simulink model "EV_mod"  (R2013b)
settings: Solver=ode1  StartTime=0.0  StopTime=tf  FixedStep=Ts  RelTol=1e-3
values from neighbouring files (symbols this model uses):
  A_Drag = 0.78    [EV_initial.m]
  Bat_Cap_Ah = 50    [EV_initial.m]
  eff_trans = 0.90    (= 0.9)    [EV_initial.m]
  f0 = 0.021    [EV_initial.m]
  f1 = 0    [EV_initial.m]
  f4 = 0    [EV_initial.m]
  g = 9.81    [EV_initial.m]
  Ki = 0.0    (= 0)    [EV_initial.m]
  Kp = 0.3    [EV_initial.m]
  m = m_Curb_WoBat_kg    (= 826)    [EV_initial.m]
  Mot_drive_n = [517 1021 2009 3247 4024 5025 6023 7017 8021 9008 10027]    [mod_tabs.mat]
  Mot_drive_ttq = [173.1 172 170.5 168.4 137.1 111.4 97.4 84.3 72.7 63.8 57.8]    [mod_tabs.mat]
  Mot_eff = [0.9093 0.9055 0.9401 0.9254 0.9287 0.9367 0.94 0.9292 0.9266 0.9191 0.8879 0.8947 ... (66 elements, 11x6)]    [mod_tabs.mat]
  R_f_charge = [0.0635340437122 0.0972918718458 0.105453801534 0.0989735084394 0.0862095416557 0.0738255704382 0.0918870144995 0.10417757919 0.0905696711114 0.0977276427179 0.0819350722889 0.155211698552 ... (16 elements, 1x16)]    [mod_tabs.mat]
  R_f_discharge = [0.12662204948 0.11936385128 0.118975090305 0.115399141433 0.117316920728 0.119061636403 0.1175114965 0.120632583027 0.128045365058 0.140195986159 0.137913717883 0.137947087219 ... (16 elements, 1x16)]    [mod_tabs.mat]
  r_gear = 9.34    [EV_initial.m]
  r_regen = 0.3    [EV_initial.m]
  SOC_f = [0.25 0.3 0.35 0.4 0.45 0.5 0.55 0.6 0.65 0.7 0.75 0.8 ... (16 elements, 1x16)]    [mod_tabs.mat]
  SOC_initial = 0.8    [EV_initial.m]
  T_brk_max = 800    [EV_initial.m]
  Uo_f_charge = [330.979042132 332.354241138 334.867975079 337.647567428 339.098272093 341.463293071 342.658764937 343.613546375 344.964982453 349.820174546 350.773879483 351.713350122 ... (16 elements, 1x16)]    [mod_tabs.mat]
  Uo_f_discharge = [329.578956913 331.264061644 334.222416797 335.977481552 337.118187606 339.421595672 340.30808504 340.898981164 343.01889846 346.179322896 346.685239696 346.505505514 ... (16 elements, 1x16)]    [mod_tabs.mat]
  v_init = v(1)/3.6    [EV_initial.m]
undefined symbols (not defined in the file): r_Wheel
libraries: simulink x1
settings Model: Creator=wanghonglei  LastModifiedBy=xinmei
settings DataIOCC: SignalLoggingSaveFormat=ModelDataLogs
settings OptimizationCC: ExpressionDepthLimit=2147483647
settings DebuggingCC: FcnCallInpInsideContextMsg=UseLocalSettings  StateNameClashWarn=warning
settings GRTTargetCC: CombineOutputUpdateFcns=off  GRTInterface=on

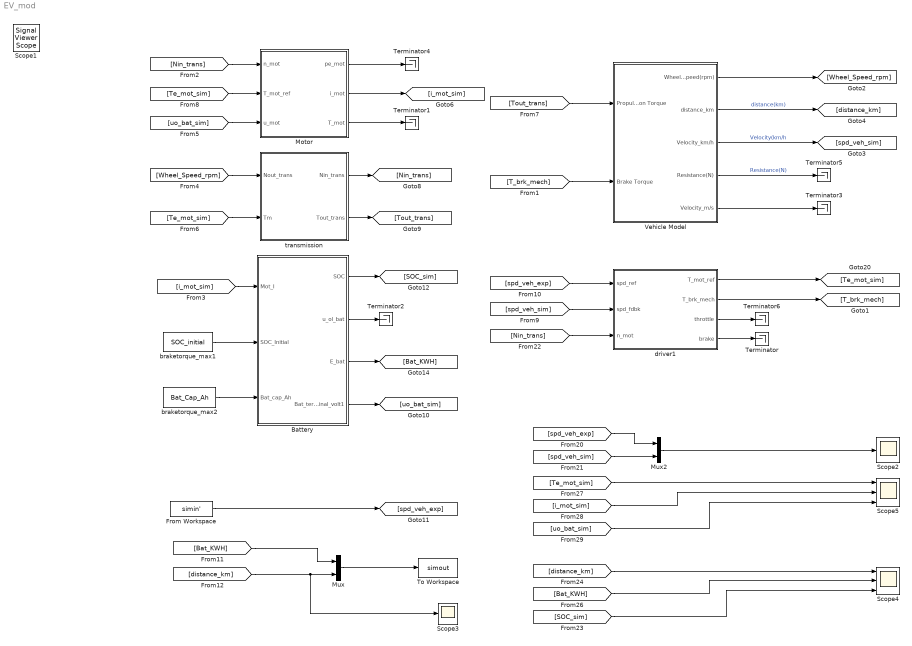
== system EV_mod ==
  Battery : Subsystem
  From Workspace : FromWorkspace  VariableName=simin'  SampleTime=0
  Motor : Subsystem
  Mux : Mux  Inputs=2
  Mux2 : Mux  Inputs=2
  Scope2 : Scope
  Scope3 : Scope
      settings: SaveName=ScopeData2
  Scope4 : Scope  NumInputPorts=3
      settings: YMin=-5~-5~-5  YMax=5~5~5  SaveName=ScopeData3
  Scope5 : Scope  NumInputPorts=3
      settings: YMin=-5~-5~-5  YMax=5~5~5
  Terminator{,1..6} (7 alike) : Terminator
  To Workspace : ToWorkspace  VariableName=simout  SampleTime=-1
      settings: MaxDataPoints=1
  Vehicle Model : Subsystem  mask{m=m, f0=f0, f1=f1, f4=f4, r=r_Wheel, A=0, K=0, g=g}
      mask prompts: m "Whole Vehicle Mass"; f0 "rolling resistant coefficient0"; f1 "rolling resistant coefficient1"; f4 "rolling resistant coefficient4"; r "radius"; A "Front Area"; K "wind resistant coeffcient"; g "Acceleration of Gravity"
  braketorque_max1 : Constant  Value=SOC_initial
  braketorque_max2 : Constant  Value=Bat_Cap_Ah
  driver1 : Subsystem
  transmission : Subsystem
  Scope1 : SignalViewerScope  IOType=viewer  NumInputPorts=4  LegendLocations=|  RefreshTime=0.035000
      | 633.2778      426.6944      187.6667         43.25
      | 712.2778      312.6944      108.6667         43.25
      | 640.2778      198.6944      180.6667         43.25
      | 640.2778      83.69444      180.6667         43.25
      settings: ShowLegends=on  TimeRange=450  YMin=0~-1~-20~-50  YMax=100~1~60~150
  wires:
  [T_brk_mech] -> Vehicle Model/2(Brake Torque)
  Vehicle Model/1(Wheel Speed(rpm)) -> [Wheel_Speed_rpm]
  [Wheel_Speed_rpm] -> transmission/1(Nout_trans)
  Vehicle Model/2(distance_km) -> [distance_km]  "distance(km)"
  transmission/1(Nin_trans) -> [Nin_trans]
  transmission/2(Tout_trans) -> [Tout_trans]
  [Tout_trans] -> Vehicle Model/1(Propulsion Torque)
  [i_mot_sim] -> Battery/1(Mot_I)
  braketorque_max1/1 -> Battery/2(SOC_Initial)
  braketorque_max2/1 -> Battery/3(Bat_cap_Ah)
  [Nin_trans] -> Motor/1(n_mot)
  Motor/2(i_mot) -> [i_mot_sim]
  [uo_bat_sim] -> Motor/3(u_mot)
  [Te_mot_sim] -> transmission/2(Tm)
  [Te_mot_sim] -> Motor/2(T_mot_ref)
  Battery/1(SOC) -> [SOC_sim]
  Battery/3(E_bat) -> [Bat_KWH]
  Battery/4(Bat_terminal_volt1) -> [uo_bat_sim]
  Battery/2(u_ol_bat) -> Terminator2/1
  Motor/1(pe_mot) -> Terminator4/1
  [spd_veh_exp] -> driver1/1(spd_ref)
  Vehicle Model/3(Velocity_km/h) -> [spd_veh_sim]  "Velocity(km/h"
  Vehicle Model/4(Resistance(N)) -> Terminator5/1  "Resistance(N)"
  Vehicle Model/5(Velocity_m/s) -> Terminator3/1
  From Workspace/1 -> [spd_veh_exp]
  [Bat_KWH] -> Mux/1
  [distance_km] -> Scope3/1, Mux/2
  Mux/1 -> To Workspace/1
  Mux2/1 -> Scope2/1
  [spd_veh_exp] -> Mux2/1
  [spd_veh_sim] -> Mux2/2
  [distance_km] -> Scope4/1
  [Bat_KWH] -> Scope4/2
  [SOC_sim] -> Scope4/3
  [Te_mot_sim] -> Scope5/1
  [i_mot_sim] -> Scope5/2
  [uo_bat_sim] -> Scope5/3
  [spd_veh_sim] -> driver1/2(spd_fdbk)
  [Nin_trans] -> driver1/3(n_mot)
  driver1/1(T_mot_ref) -> [Te_mot_sim]
  driver1/2(T_brk_mech) -> [T_brk_mech]
  driver1/3(throttle) -> Terminator6/1
  driver1/4(brake) -> Terminator/1
  Motor/3(T_mot) -> Terminator1/1

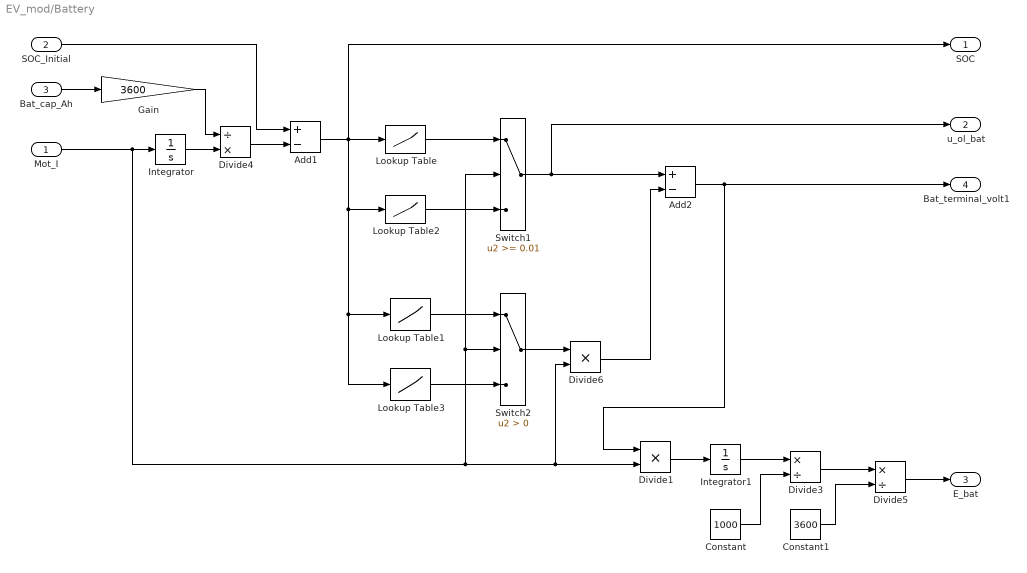
== system EV_mod/Battery ==
  Mot_I : Inport
  SOC_Initial : Inport  Port=2
  Bat_cap_Ah : Inport  Port=3
  Add1 : Sum  Inputs=+-
  Add2 : Sum  Inputs=+-
  Constant : Constant  Value=1000
  Constant1 : Constant  Value=3600
  Divide1 : Product  Inputs=**
  Divide3 : Product  Inputs=*/
  Divide4 : Product  Inputs=/*
  Divide5 : Product  Inputs=*/
  Divide6 : Product  Inputs=**
  Gain : Gain  Gain=3600
  Integrator : Integrator
  Integrator1 : Integrator
  Lookup Table : Lookup  InputValues=SOC_f  Table=Uo_f_discharge
  Lookup Table1 : Lookup  InputValues=SOC_f  Table=R_f_discharge
  Lookup Table2 : Lookup  InputValues=SOC_f  Table=Uo_f_charge
  Lookup Table3 : Lookup  InputValues=SOC_f  Table=R_f_charge
  Switch1 : Switch  Threshold=0.01
  Switch2 : Switch  Criteria=u2 > Threshold
  SOC : Outport
  u_ol_bat : Outport  Port=2
  E_bat : Outport  Port=3
  Bat_terminal_volt1 : Outport  Port=4
  wires:
  Bat_cap_Ah/1 -> Gain/1
  SOC_Initial/1 -> Add1/1
  Divide1/1 -> Integrator1/1
  Integrator1/1 -> Divide3/1
  Constant/1 -> Divide3/2
  Divide3/1 -> Divide5/1
  Constant1/1 -> Divide5/2
  Divide5/1 -> E_bat/1
  Divide6/1 -> Add2/2
  Add1/1 -> Lookup Table/1, Lookup Table3/1, Lookup Table1/1, Lookup Table2/1, SOC/1
  Switch2/1 -> Divide6/1
  Switch1/1 -> u_ol_bat/1, Add2/1
  Lookup Table/1 -> Switch1/1
  Lookup Table2/1 -> Switch1/3
  Mot_I/1 -> Switch2/2, Switch1/2, Divide6/2, Divide1/2, Integrator/1
  Lookup Table3/1 -> Switch2/3
  Lookup Table1/1 -> Switch2/1
  Add2/1 -> Bat_terminal_volt1/1, Divide1/1
  Integrator/1 -> Divide4/2
  Gain/1 -> Divide4/1
  Divide4/1 -> Add1/2

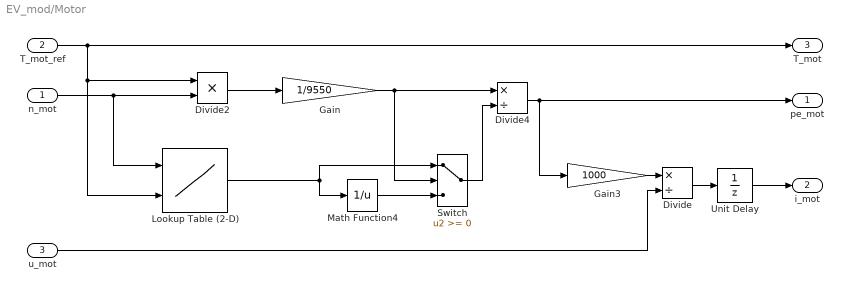
== system EV_mod/Motor ==
  n_mot : Inport
  T_mot_ref : Inport  Port=2
  u_mot : Inport  Port=3
  Divide : Product  Inputs=*/
  Divide2 : Product  Inputs=**
  Divide4 : Product  Inputs=*/
  Gain : Gain  Gain=1/9550
  Gain3 : Gain  Gain=1000
  Lookup Table (2-D) : Lookup2D  RowIndex=Mot_eff_n  ColumnIndex=Mot_eff_ttq  Table=Mot_eff  LookUpMeth=Interpolation-Use End Values
  Math Function4 : Math  Operator=reciprocal  SaturateOnIntegerOverflow=on
  Switch : Switch
  Unit Delay : UnitDelay  SampleTime=-1
  pe_mot : Outport
  i_mot : Outport  Port=2
  T_mot : Outport  Port=3
  wires:
  Divide2/1 -> Gain/1
  Switch/1 -> Divide4/2
  Divide4/1 -> pe_mot/1, Gain3/1
  u_mot/1 -> Divide/2
  Divide/1 -> Unit Delay/1
  Gain3/1 -> Divide/1
  Gain/1 -> Switch/2, Divide4/1
  Lookup Table (2-D)/1 -> Math Function4/1, Switch/1
  Math Function4/1 -> Switch/3
  Unit Delay/1 -> i_mot/1
  n_mot/1 -> Lookup Table (2-D)/1, Divide2/2
  T_mot_ref/1 -> T_mot/1, Lookup Table (2-D)/2, Divide2/1

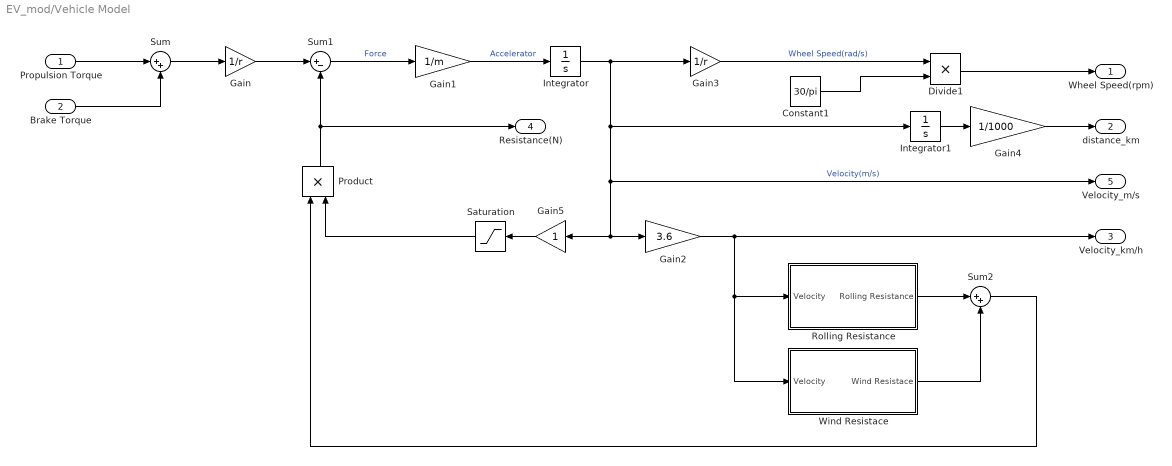
== system EV_mod/Vehicle Model ==
  Propulsion Torque : Inport
  Brake Torque : Inport  Port=2
  Constant1 : Constant  Value=30/pi
  Divide1 : Product  Inputs=**
  Gain : Gain  Gain=1/r
  Gain1 : Gain  Gain=1/m
  Gain2 : Gain  Gain=3.6
  Gain3 : Gain  Gain=1/r
  Gain4 : Gain  Gain=1/1000
  Gain5 : Gain
  Integrator : Integrator  InitialCondition=v_init
  Integrator1 : Integrator
  Product : Product  RndMeth=Zero
  Rolling Resistance : Subsystem
  Saturation : Saturate  UpperLimit=1  LowerLimit=-1
  Sum : Sum  Inputs=|++
  Sum1 : Sum  Inputs=|+-
  Sum2 : Sum  Inputs=|++
  Wind Resistace : Subsystem
  Wheel Speed(rpm) : Outport
  distance_km : Outport  Port=2
  Velocity_km/h : Outport  Port=3
  Resistance(N) : Outport  Port=4
  Velocity_m/s : Outport  Port=5
  wires:
  Propulsion Torque/1 -> Sum/1
  Brake Torque/1 -> Sum/2
  Sum/1 -> Gain/1
  Gain/1 -> Sum1/1
  Sum1/1 -> Gain1/1  "Force"
  Gain1/1 -> Integrator/1  "Accelerator"
  Integrator/1 -> Gain5/1, Gain2/1, Velocity_m/s/1, Integrator1/1, Gain3/1  "Velocity(m/s)"
  Integrator1/1 -> Gain4/1
  Gain4/1 -> distance_km/1
  Rolling Resistance/1(Rolling Resistance) -> Sum2/1
  Wind Resistace/1(Wind Resistace) -> Sum2/2
  Gain2/1 -> Velocity_km/h/1, Rolling Resistance/1(Velocity), Wind Resistace/1(Velocity)
  Sum2/1 -> Product/1
  Gain5/1 -> Saturation/1
  Saturation/1 -> Product/2
  Product/1 -> Resistance(N)/1, Sum1/2
  Constant1/1 -> Divide1/2
  Gain3/1 -> Divide1/1  "Wheel Speed(rad/s)"
  Divide1/1 -> Wheel Speed(rpm)/1

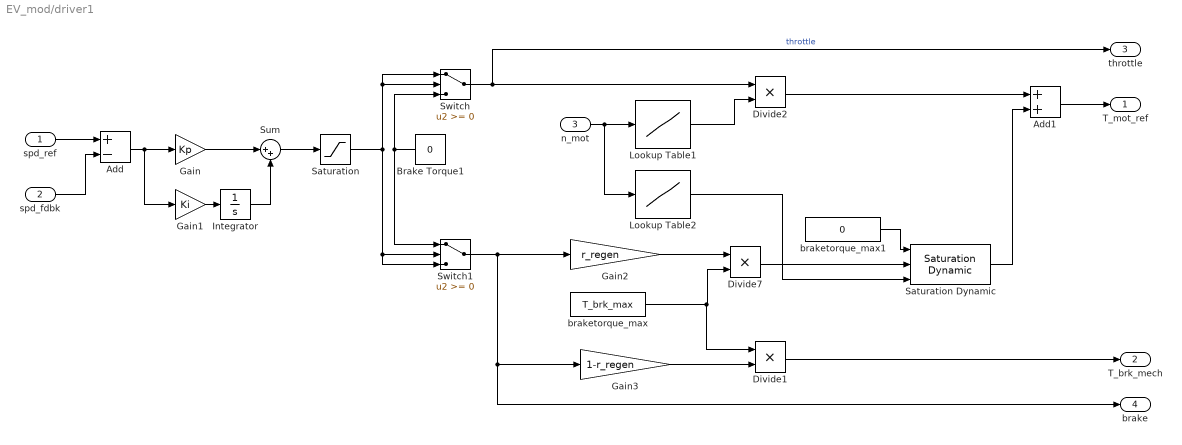
== system EV_mod/driver1 ==
  spd_ref : Inport
  spd_fdbk : Inport  Port=2
  n_mot : Inport  Port=3
  Add : Sum  Inputs=+-
  Add1 : Sum
  Brake Torque1 : Constant  Value=0
  Divide1 : Product  Inputs=**
  Divide2 : Product  Inputs=**
  Divide7 : Product  Inputs=**
  Gain : Gain  Gain=Kp
  Gain1 : Gain  Gain=Ki
  Gain2 : Gain  Gain=r_regen
  Gain3 : Gain  Gain=1-r_regen
  Integrator : Integrator
  Lookup Table1 : Lookup  InputValues=Mot_drive_n  Table=Mot_drive_ttq
  Lookup Table2 : Lookup  InputValues=Mot_drive_n  Table=-Mot_drive_ttq
  Saturation : Saturate  UpperLimit=1  LowerLimit=-1
  Saturation Dynamic : simulink/Discontinuities/Saturation Dynamic  OutMin=[]  OutMax=[]  OutDataTypeStr=Inherit: Same as second input  OutDataType=fixdt(1, 16)  OutScaling=2^-10  DoSatur=off
  Sum : Sum  Inputs=|++
  Switch : Switch
  Switch1 : Switch
  braketorque_max : Constant  Value=T_brk_max
  braketorque_max1 : Constant  Value=0
  T_mot_ref : Outport
  T_brk_mech : Outport  Port=2
  throttle : Outport  Port=3
  brake : Outport  Port=4
  wires:
  spd_ref/1 -> Add/1
  Brake Torque1/1 -> Switch/3, Switch1/1
  Saturation/1 -> Switch/1, Switch/2, Switch1/2, Switch1/3
  Add/1 -> Gain1/1, Gain/1
  Gain/1 -> Sum/1
  Sum/1 -> Saturation/1
  Gain1/1 -> Integrator/1
  Integrator/1 -> Sum/2
  spd_fdbk/1 -> Add/2
  Switch/1 -> Divide2/1, throttle/1  "throttle"
  Switch1/1 -> Gain2/1, Gain3/1, brake/1
  n_mot/1 -> Lookup Table2/1, Lookup Table1/1
  Divide2/1 -> Add1/1
  Gain2/1 -> Divide7/1
  braketorque_max/1 -> Divide1/1, Divide7/2
  Divide7/1 -> Saturation Dynamic/2
  Saturation Dynamic/1 -> Add1/2
  Add1/1 -> T_mot_ref/1
  Gain3/1 -> Divide1/2
  Divide1/1 -> T_brk_mech/1
  braketorque_max1/1 -> Saturation Dynamic/1
  Lookup Table2/1 -> Saturation Dynamic/3
  Lookup Table1/1 -> Divide2/2

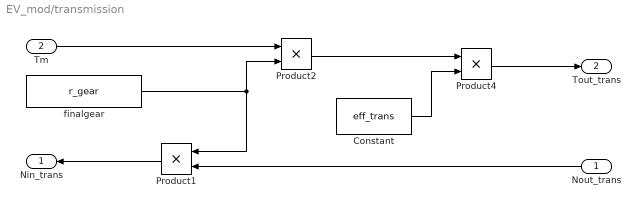
== system EV_mod/transmission ==
  Nout_trans : Inport
  Tm : Inport  Port=2
  Constant : Constant  Value=eff_trans
  Product1 : Product  RndMeth=Zero
  Product2 : Product  RndMeth=Zero
  Product4 : Product  RndMeth=Zero
  finalgear : Constant  Value=r_gear
  Nin_trans : Outport
  Tout_trans : Outport  Port=2
  wires:
  Nout_trans/1 -> Product1/2
  Product2/1 -> Product4/1
  Constant/1 -> Product4/2
  Product4/1 -> Tout_trans/1
  finalgear/1 -> Product2/2, Product1/1
  Tm/1 -> Product2/1
  Product1/1 -> Nin_trans/1

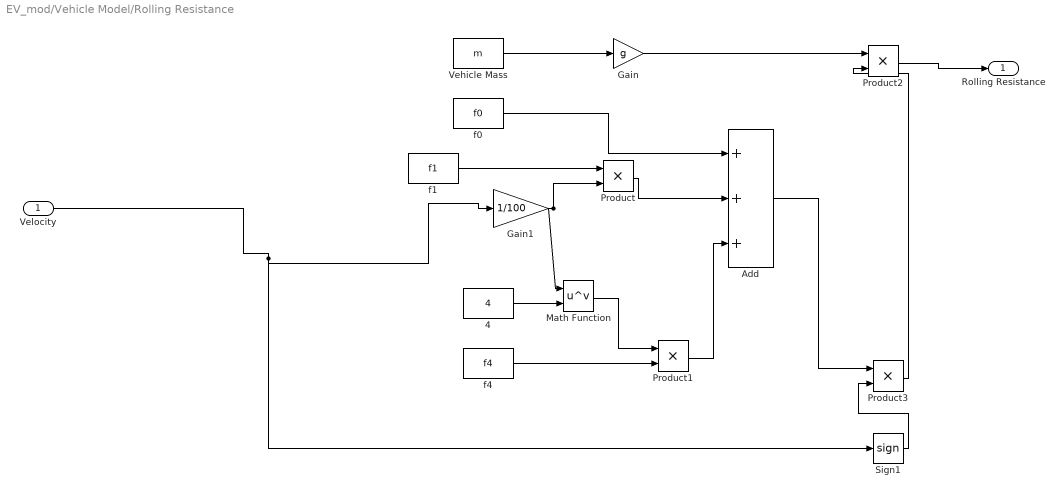
== system EV_mod/Vehicle Model/Rolling Resistance ==
  Velocity : Inport
  4 : Constant  Value=4
  Add : Sum  Inputs=+++
  Gain : Gain  Gain=g
  Gain1 : Gain  Gain=1/100
  Math Function : Math  Operator=pow  SaturateOnIntegerOverflow=on
  Product{,1..3} (4 alike) : Product  RndMeth=Zero
  Sign1 : Signum
  Vehicle Mass : Constant  Value=m
  f0 : Constant  Value=f0
  f1 : Constant  Value=f1
  f4 : Constant  Value=f4
  Rolling Resistance : Outport
  wires:
  Vehicle Mass/1 -> Gain/1
  f0/1 -> Add/1
  Gain1/1 -> Product/2, Math Function/1
  Product/1 -> Add/2
  4/1 -> Math Function/2
  Math Function/1 -> Product1/1
  f4/1 -> Product1/2
  Product1/1 -> Add/3
  Gain/1 -> Product2/1
  Product2/1 -> Rolling Resistance/1
  f1/1 -> Product/1
  Velocity/1 -> Gain1/1, Sign1/1
  Add/1 -> Product3/1
  Sign1/1 -> Product3/2
  Product3/1 -> Product2/2

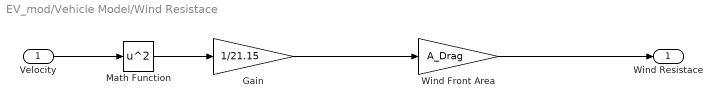
== system EV_mod/Vehicle Model/Wind Resistace ==
  Velocity : Inport
  Gain : Gain  Gain=1/21.15
  Math Function : Math  Operator=square  SaturateOnIntegerOverflow=on
  Wind Front Area : Gain  Gain=A_Drag
  Wind Resistace : Outport
  wires:
  Velocity/1 -> Math Function/1
  Math Function/1 -> Gain/1
  Gain/1 -> Wind Front Area/1
  Wind Front Area/1 -> Wind Resistace/1
